simulink model "SLS_ChainModel_Sim"  (R2025a)
settings: Solver=VariableStepAuto  StartTime=0.0  StopTime=50  FixedStep=1e-3  RelTol=1e-3
values from neighbouring files (symbols this model uses):
  Phiu1 = full(Phiu{1})    [Distributed_Sim.m]
  Phiu2 = full(Phiu{2})    [Distributed_Sim.m]
  Phiu3 = full(Phiu{3})    [Distributed_Sim.m]
  Phiu4 = full(Phiu{4})    [Distributed_Sim.m]
  Phix1 = full(Phix{1})    [Distributed_Sim.m]
  Phix2 = full(Phix{2})    [Distributed_Sim.m]
  Phix3 = full(Phix{3})    [Distributed_Sim.m]
  Phix4 = full(Phix{4})    [Distributed_Sim.m]
  slsp1 = SLSPoles(1)    [Distributed_Sim.m]
  slsp2 = SLSPoles(2)    [Distributed_Sim.m]
  slsp3 = SLSPoles(3)    [Distributed_Sim.m]
  slsp4 = SLSPoles(4)    [Distributed_Sim.m]
  sysA = sys.A    [Distributed_Sim.m]    (also in Simple_Poles_Hinf.m = powersys.A; grid_model.mat = )
  sysB = sys.B2    [Distributed_Sim.m]    (also in Simple_Poles_Hinf.m = powersys.B2; grid_model.mat = )
undefined symbols (not defined in the file or in its folder): full
settings Model: Creator=johnd  LastModifiedBy=johnd
settings RTWCC: GPUComputeCapability=3.5

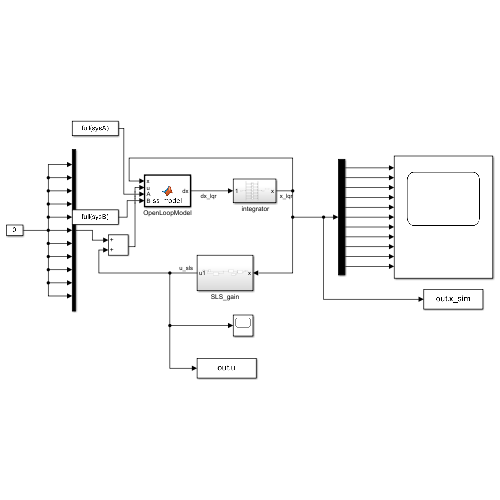
[thumbnail: Simulink's stored preview of the top-level diagram]
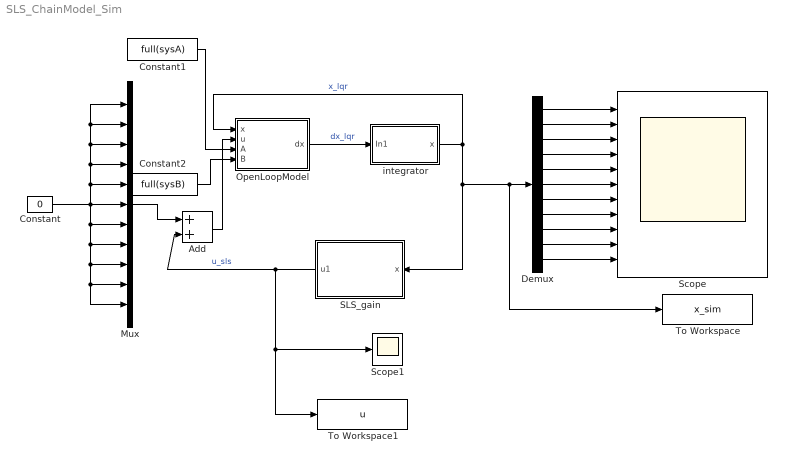
== system SLS_ChainModel_Sim ==
  " integrator" : Subsystem
  Add : Sum
  Constant : Constant  Value=0
  Constant1 : Constant  Value=full(sysA)
  Constant2 : Constant  Value=full(sysB)
  Demux : Demux  Outputs=11
  Mux : Mux  Inputs=11
  OpenLoopModel : MATLAB Function  TreatAsAtomicUnit=on
  SLS_gain : Subsystem
  Scope : Scope  NumInputPorts=11
      settings: ActiveDisplayYMinimum=-2.9E-35  ActiveDisplayYMaximum=3E-36
  Scope1 : Scope
      settings: ActiveDisplayYMinimum=-2.09753  ActiveDisplayYMaximum=0.3482
  To Workspace : ToWorkspace  VariableName=x_sim  SaveFormat=Timeseries  SampleTime=-1
  To Workspace1 : ToWorkspace  VariableName=u  SaveFormat=Timeseries  SampleTime=-1
  wires:
  OpenLoopModel/1(dx) -> " integrator"/1(In1)  "dx_lqr"
  " integrator"/1(x) -> SLS_gain/1(x), To Workspace/1, Demux/1, OpenLoopModel/1(x)  "x_lqr"
  Constant/1 -> Mux/6, Mux/7, Mux/8, Mux/9, Mux/10, Mux/11, Mux/5, Mux/4, Mux/3, Mux/2, Mux/1
  SLS_gain/1(u1) -> To Workspace1/1, Scope1/1, Add/2  "u_sls"
  Mux/1 -> Add/1
  Add/1 -> OpenLoopModel/2(u)
  Demux/1 -> Scope/1
  Demux/3 -> Scope/3
  Demux/2 -> Scope/2
  Demux/4 -> Scope/4
  Demux/5 -> Scope/5
  Demux/6 -> Scope/6
  Demux/7 -> Scope/7
  Demux/8 -> Scope/8
  Demux/9 -> Scope/9
  Demux/10 -> Scope/10
  Demux/11 -> Scope/11
  Constant1/1 -> OpenLoopModel/3(A)
  Constant2/1 -> OpenLoopModel/4(B)

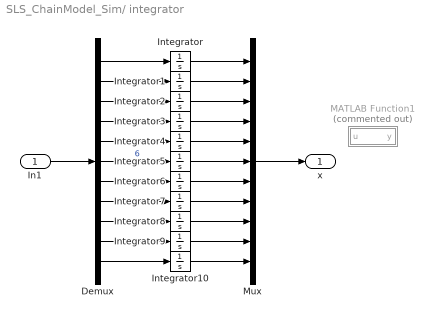
== system SLS_ChainModel_Sim/ integrator ==
  In1 : Inport
  Demux : Demux  Outputs=11
  Integrator{,1..4,6..10} (10 alike) : Integrator
  Integrator5 : Integrator  InitialCondition=1
  MATLAB Function1 : MATLAB Function  Commented=on  TreatAsAtomicUnit=on
  Mux : Mux  Inputs=11
  x : Outport
  wires:
  Demux/1 -> Integrator/1
  Demux/2 -> Integrator1/1
  Mux/1 -> x/1
  In1/1 -> Demux/1
  Demux/3 -> Integrator2/1
  Demux/4 -> Integrator3/1
  Demux/5 -> Integrator4/1
  Demux/6 -> Integrator5/1  "6"
  Demux/7 -> Integrator6/1
  Demux/8 -> Integrator7/1
  Demux/9 -> Integrator8/1
  Demux/10 -> Integrator9/1
  Demux/11 -> Integrator10/1
  Integrator/1 -> Mux/1
  Integrator1/1 -> Mux/2
  Integrator2/1 -> Mux/3
  Integrator3/1 -> Mux/4
  Integrator4/1 -> Mux/5
  Integrator5/1 -> Mux/6
  Integrator6/1 -> Mux/7
  Integrator7/1 -> Mux/8
  Integrator8/1 -> Mux/9
  Integrator9/1 -> Mux/10
  Integrator10/1 -> Mux/11

== system SLS_ChainModel_Sim/SLS_gain ==
  x : Inport
  Constant : Constant  Value=full(sysB)
  MATLAB Function : MATLAB Function  TreatAsAtomicUnit=on
  S*Phi_u(s)1 : Subsystem
  S*Phi_x(s) : Subsystem
  Subtract1 : Sum  Inputs=+-
  u1 : Outport
  wires:
  Subtract1/1 -> S*Phi_u(s)1/1(I), S*Phi_x(s)/1(v)  "v"
  x/1 -> Subtract1/1
  S*Phi_x(s)/1((s*phi_x(s)-I)) -> Subtract1/2
  S*Phi_u(s)1/1(s*phi_u(s)) -> MATLAB Function/1(u)
  MATLAB Function/1(y) -> u1/1
  Constant/1 -> MATLAB Function/2(B)

== system SLS_ChainModel_Sim/SLS_gain/S*Phi_u(s)1 ==
  note: This is for a 2-poles system
  I : Inport
  Add : Sum
  Pair1 : Subsystem
  Pair2 : Subsystem
  s*phi_u(s) : Outport
  wires:
  I/1 -> Pair2/1(u), Pair1/1(u)
  Pair1/1(s*phi_u(s)) -> Add/1
  Add/1 -> s*phi_u(s)/1
  Pair2/1(s*phi_u(s)) -> Add/2

== system SLS_ChainModel_Sim/SLS_gain/S*Phi_x(s) ==
  note: This is for a 2-poles system
  v : Inport
  Add : Sum
  Pair1 : Subsystem
  Pair2 : Subsystem
  (s*phi_x(s)-I) : Outport
  wires:
  v/1 -> Pair1/1(In1), Pair2/1(v)
  Pair1/1(Out1) -> Add/1
  Pair2/1(Out1) -> Add/2
  Add/1 -> (s*phi_x(s)-I)/1

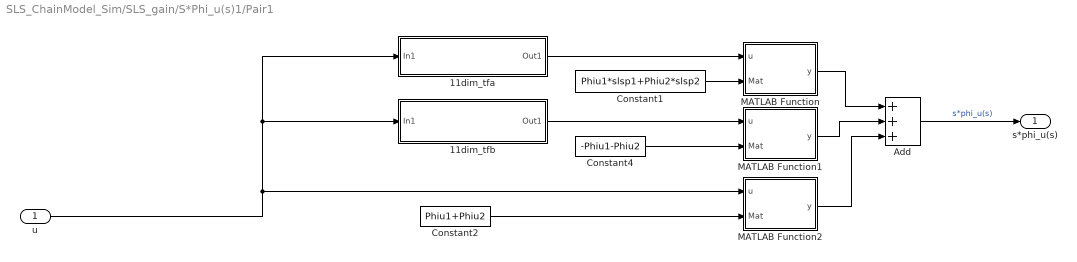
== system SLS_ChainModel_Sim/SLS_gain/S*Phi_u(s)1/Pair1 ==
  u : Inport
  11dim_tfa : Subsystem
  11dim_tfb : Subsystem
  Add : Sum  Inputs=+++
  Constant1 : Constant  Value=Phiu1*slsp1+Phiu2*slsp2  VectorParams1D=off
  Constant2 : Constant  Value=Phiu1+Phiu2
  Constant4 : Constant  Value=-Phiu1-Phiu2
  MATLAB Function : MATLAB Function  TreatAsAtomicUnit=on
  MATLAB Function1 : MATLAB Function  TreatAsAtomicUnit=on
  MATLAB Function2 : MATLAB Function  TreatAsAtomicUnit=on
  s*phi_u(s) : Outport
  wires:
  MATLAB Function/1(y) -> Add/1
  u/1 -> 11dim_tfb/1(In1), 11dim_tfa/1(In1), MATLAB Function2/1(u)
  11dim_tfa/1(Out1) -> MATLAB Function/1(u)
  MATLAB Function1/1(y) -> Add/2
  11dim_tfb/1(Out1) -> MATLAB Function1/1(u)
  MATLAB Function2/1(y) -> Add/3
  Constant1/1 -> MATLAB Function/2(Mat)
  Constant2/1 -> MATLAB Function2/2(Mat)
  Constant4/1 -> MATLAB Function1/2(Mat)
  Add/1 -> s*phi_u(s)/1  "s*phi_u(s)"

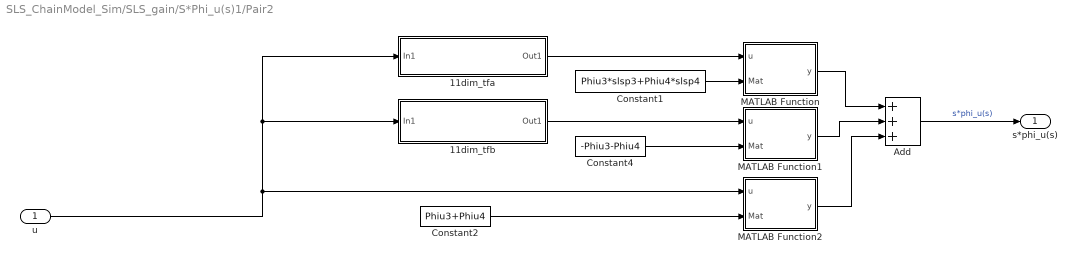
== system SLS_ChainModel_Sim/SLS_gain/S*Phi_u(s)1/Pair2 ==
  u : Inport
  11dim_tfa : Subsystem
  11dim_tfb : Subsystem
  Add : Sum  Inputs=+++
  Constant1 : Constant  Value=Phiu3*slsp3+Phiu4*slsp4  VectorParams1D=off
  Constant2 : Constant  Value=Phiu3+Phiu4
  Constant4 : Constant  Value=-Phiu3-Phiu4
  MATLAB Function : MATLAB Function  TreatAsAtomicUnit=on
  MATLAB Function1 : MATLAB Function  TreatAsAtomicUnit=on
  MATLAB Function2 : MATLAB Function  TreatAsAtomicUnit=on
  s*phi_u(s) : Outport
  wires:
  Add/1 -> s*phi_u(s)/1  "s*phi_u(s)"
  Constant4/1 -> MATLAB Function1/2(Mat)
  Constant2/1 -> MATLAB Function2/2(Mat)
  Constant1/1 -> MATLAB Function/2(Mat)
  MATLAB Function2/1(y) -> Add/3
  11dim_tfb/1(Out1) -> MATLAB Function1/1(u)
  MATLAB Function1/1(y) -> Add/2
  11dim_tfa/1(Out1) -> MATLAB Function/1(u)
  u/1 -> MATLAB Function2/1(u), 11dim_tfa/1(In1), 11dim_tfb/1(In1)
  MATLAB Function/1(y) -> Add/1

== system SLS_ChainModel_Sim/SLS_gain/S*Phi_x(s)/Pair1 ==
  In1 : Inport
  11dim_tfa : Subsystem
  11dim_tfb : Subsystem
  Add : Sum
  Constant1 : Constant  Value=Phix1*slsp1+Phix2*slsp2
  Constant4 : Constant  Value=-Phix1-Phix2
  MATLAB Function : MATLAB Function  TreatAsAtomicUnit=on
  MATLAB Function1 : MATLAB Function  TreatAsAtomicUnit=on
  Out1 : Outport
  wires:
  Add/1 -> Out1/1
  MATLAB Function/1(y) -> Add/1
  11dim_tfb/1(Out1) -> MATLAB Function1/1(u)
  In1/1 -> 11dim_tfa/1(In1), 11dim_tfb/1(In1)
  11dim_tfa/1(Out1) -> MATLAB Function/1(u)
  MATLAB Function1/1(y) -> Add/2
  Constant1/1 -> MATLAB Function/2(Mat)
  Constant4/1 -> MATLAB Function1/2(Mat)

== system SLS_ChainModel_Sim/SLS_gain/S*Phi_x(s)/Pair2 ==
  v : Inport
  11dim_tfa : Subsystem
  11dim_tfb : Subsystem
  Add : Sum
  Constant1 : Constant  Value=Phix3*slsp3+Phix4*slsp4
  Constant4 : Constant  Value=-Phix3-Phix4
  MATLAB Function : MATLAB Function  TreatAsAtomicUnit=on
  MATLAB Function1 : MATLAB Function  TreatAsAtomicUnit=on
  Out1 : Outport
  wires:
  Constant4/1 -> MATLAB Function1/2(Mat)
  Constant1/1 -> MATLAB Function/2(Mat)
  MATLAB Function1/1(y) -> Add/2
  11dim_tfa/1(Out1) -> MATLAB Function/1(u)
  v/1 -> 11dim_tfb/1(In1), 11dim_tfa/1(In1)
  11dim_tfb/1(Out1) -> MATLAB Function1/1(u)
  MATLAB Function/1(y) -> Add/1
  Add/1 -> Out1/1

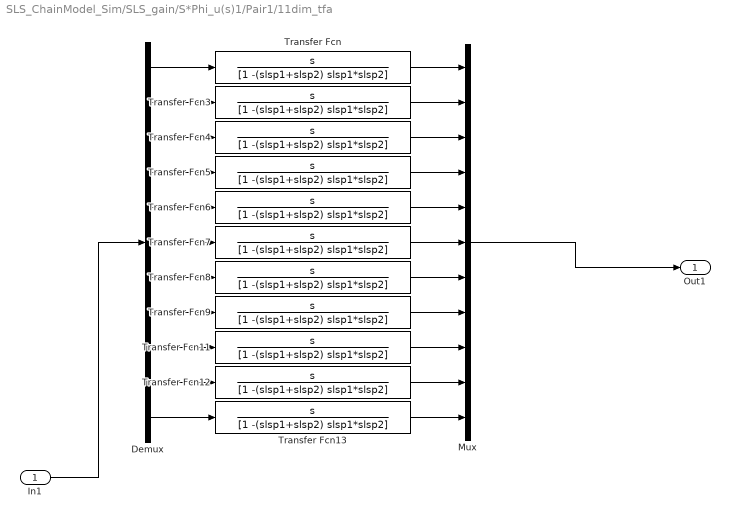
== system SLS_ChainModel_Sim/SLS_gain/S*Phi_u(s)1/Pair1/11dim_tfa ==
  In1 : Inport
  Demux : Demux  Outputs=11
  Mux : Mux  Inputs=11
  Transfer Fcn{,3..9,11..13} (11 alike) : TransferFcn  Numerator=[0 1 0]  Denominator=[1 -(slsp1+slsp2) slsp1*slsp2]
  Out1 : Outport
  wires:
  Transfer Fcn12/1 -> Mux/10
  Demux/7 -> Transfer Fcn8/1
  Transfer Fcn7/1 -> Mux/6
  Demux/4 -> Transfer Fcn5/1
  Demux/2 -> Transfer Fcn3/1
  Demux/9 -> Transfer Fcn11/1
  In1/1 -> Demux/1
  Transfer Fcn9/1 -> Mux/8
  Demux/10 -> Transfer Fcn12/1
  Demux/6 -> Transfer Fcn7/1
  Demux/11 -> Transfer Fcn13/1
  Demux/8 -> Transfer Fcn9/1
  Transfer Fcn11/1 -> Mux/9
  Transfer Fcn5/1 -> Mux/4
  Transfer Fcn3/1 -> Mux/2
  Transfer Fcn4/1 -> Mux/3
  Transfer Fcn6/1 -> Mux/5
  Demux/5 -> Transfer Fcn6/1
  Mux/1 -> Out1/1
  Demux/3 -> Transfer Fcn4/1
  Transfer Fcn8/1 -> Mux/7
  Transfer Fcn13/1 -> Mux/11
  Demux/1 -> Transfer Fcn/1
  Transfer Fcn/1 -> Mux/1

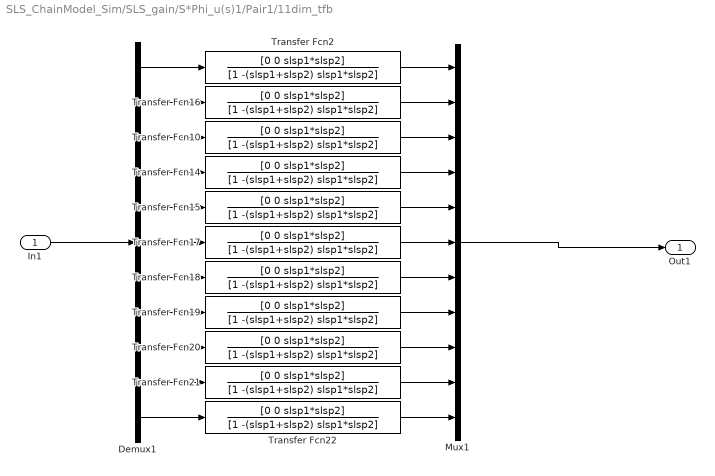
== system SLS_ChainModel_Sim/SLS_gain/S*Phi_u(s)1/Pair1/11dim_tfb ==
  In1 : Inport
  Demux1 : Demux  Outputs=11
  Mux1 : Mux  Inputs=11
  Transfer Fcn{2,10,14..22} (11 alike) : TransferFcn  Numerator=[0 0 slsp1*slsp2]  Denominator=[1 -(slsp1+slsp2) slsp1*slsp2]
  Out1 : Outport
  wires:
  Transfer Fcn20/1 -> Mux1/9
  Demux1/8 -> Transfer Fcn19/1
  Transfer Fcn18/1 -> Mux1/7
  Demux1/7 -> Transfer Fcn18/1
  Transfer Fcn19/1 -> Mux1/8
  Demux1/11 -> Transfer Fcn22/1
  Demux1/4 -> Transfer Fcn14/1
  Transfer Fcn16/1 -> Mux1/2
  Demux1/3 -> Transfer Fcn10/1
  Transfer Fcn10/1 -> Mux1/3
  Demux1/2 -> Transfer Fcn16/1
  Demux1/9 -> Transfer Fcn20/1
  Demux1/10 -> Transfer Fcn21/1
  Transfer Fcn2/1 -> Mux1/1
  Transfer Fcn22/1 -> Mux1/11
  Demux1/1 -> Transfer Fcn2/1
  Demux1/5 -> Transfer Fcn15/1
  In1/1 -> Demux1/1
  Mux1/1 -> Out1/1
  Transfer Fcn15/1 -> Mux1/5
  Demux1/6 -> Transfer Fcn17/1
  Transfer Fcn17/1 -> Mux1/6
  Transfer Fcn14/1 -> Mux1/4
  Transfer Fcn21/1 -> Mux1/10

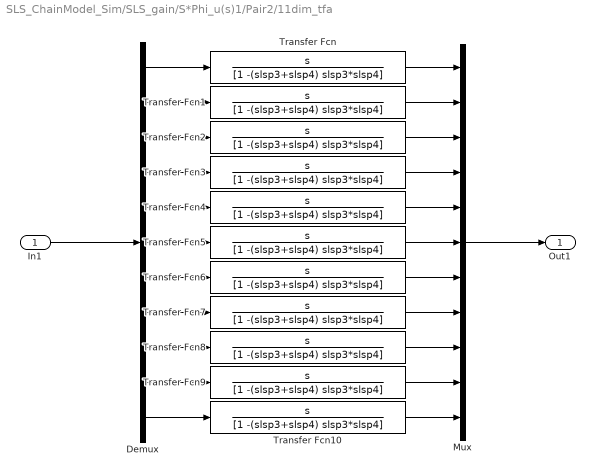
== system SLS_ChainModel_Sim/SLS_gain/S*Phi_u(s)1/Pair2/11dim_tfa ==
  In1 : Inport
  Demux : Demux  Outputs=11
  Mux : Mux  Inputs=11
  Transfer Fcn{,1..10} (11 alike) : TransferFcn  Numerator=[0 1 0]  Denominator=[1 -(slsp3+slsp4) slsp3*slsp4]
  Out1 : Outport
  wires:
  Transfer Fcn/1 -> Mux/1
  Demux/1 -> Transfer Fcn/1
  Transfer Fcn10/1 -> Mux/11
  Transfer Fcn6/1 -> Mux/7
  Demux/3 -> Transfer Fcn2/1
  Mux/1 -> Out1/1
  Demux/5 -> Transfer Fcn4/1
  Transfer Fcn4/1 -> Mux/5
  Transfer Fcn2/1 -> Mux/3
  Transfer Fcn1/1 -> Mux/2
  Transfer Fcn3/1 -> Mux/4
  Transfer Fcn8/1 -> Mux/9
  Demux/8 -> Transfer Fcn7/1
  Demux/11 -> Transfer Fcn10/1
  Demux/6 -> Transfer Fcn5/1
  Demux/10 -> Transfer Fcn9/1
  Transfer Fcn7/1 -> Mux/8
  In1/1 -> Demux/1
  Demux/9 -> Transfer Fcn8/1
  Demux/2 -> Transfer Fcn1/1
  Demux/4 -> Transfer Fcn3/1
  Transfer Fcn5/1 -> Mux/6
  Demux/7 -> Transfer Fcn6/1
  Transfer Fcn9/1 -> Mux/10

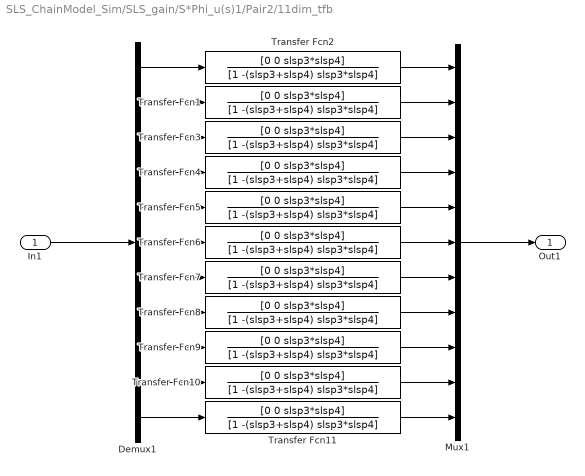
== system SLS_ChainModel_Sim/SLS_gain/S*Phi_u(s)1/Pair2/11dim_tfb ==
  In1 : Inport
  Demux1 : Demux  Outputs=11
  Mux1 : Mux  Inputs=11
  Transfer Fcn{1..11} (11 alike) : TransferFcn  Numerator=[0 0 slsp3*slsp4]  Denominator=[1 -(slsp3+slsp4) slsp3*slsp4]
  Out1 : Outport
  wires:
  Transfer Fcn10/1 -> Mux1/10
  Transfer Fcn4/1 -> Mux1/4
  Transfer Fcn6/1 -> Mux1/6
  Demux1/6 -> Transfer Fcn6/1
  Transfer Fcn5/1 -> Mux1/5
  Mux1/1 -> Out1/1
  In1/1 -> Demux1/1
  Demux1/5 -> Transfer Fcn5/1
  Demux1/1 -> Transfer Fcn2/1
  Transfer Fcn11/1 -> Mux1/11
  Transfer Fcn2/1 -> Mux1/1
  Demux1/10 -> Transfer Fcn10/1
  Demux1/9 -> Transfer Fcn9/1
  Demux1/2 -> Transfer Fcn1/1
  Transfer Fcn3/1 -> Mux1/3
  Demux1/3 -> Transfer Fcn3/1
  Transfer Fcn1/1 -> Mux1/2
  Demux1/4 -> Transfer Fcn4/1
  Demux1/11 -> Transfer Fcn11/1
  Transfer Fcn8/1 -> Mux1/8
  Demux1/7 -> Transfer Fcn7/1
  Transfer Fcn7/1 -> Mux1/7
  Demux1/8 -> Transfer Fcn8/1
  Transfer Fcn9/1 -> Mux1/9

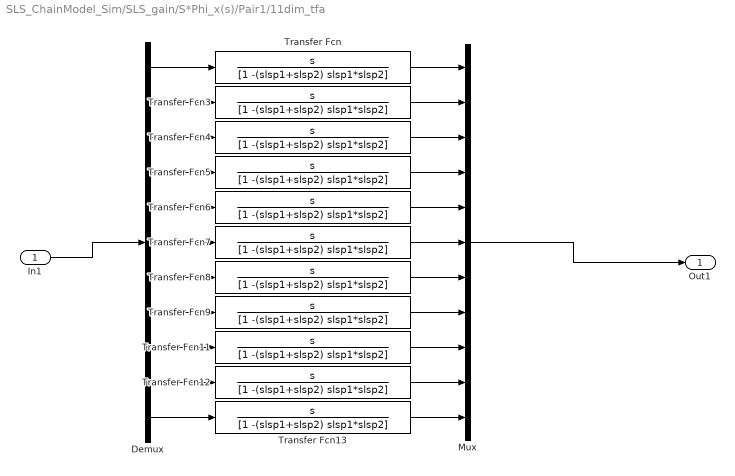
== system SLS_ChainModel_Sim/SLS_gain/S*Phi_x(s)/Pair1/11dim_tfa ==
  In1 : Inport
  Demux : Demux  Outputs=11
  Mux : Mux  Inputs=11
  Transfer Fcn{,3..9,11..13} (11 alike) : TransferFcn  Numerator=[0 1 0]  Denominator=[1 -(slsp1+slsp2) slsp1*slsp2]
  Out1 : Outport
  wires:
  Transfer Fcn13/1 -> Mux/11
  Transfer Fcn3/1 -> Mux/2
  Demux/5 -> Transfer Fcn6/1
  Demux/1 -> Transfer Fcn/1
  Transfer Fcn4/1 -> Mux/3
  Demux/7 -> Transfer Fcn8/1
  Transfer Fcn8/1 -> Mux/7
  Transfer Fcn6/1 -> Mux/5
  Transfer Fcn/1 -> Mux/1
  Demux/2 -> Transfer Fcn3/1
  Demux/8 -> Transfer Fcn9/1
  Transfer Fcn11/1 -> Mux/9
  Demux/3 -> Transfer Fcn4/1
  Transfer Fcn12/1 -> Mux/10
  Demux/11 -> Transfer Fcn13/1
  Transfer Fcn7/1 -> Mux/6
  Transfer Fcn9/1 -> Mux/8
  Demux/6 -> Transfer Fcn7/1
  Demux/4 -> Transfer Fcn5/1
  Demux/10 -> Transfer Fcn12/1
  Mux/1 -> Out1/1
  Transfer Fcn5/1 -> Mux/4
  Demux/9 -> Transfer Fcn11/1
  In1/1 -> Demux/1

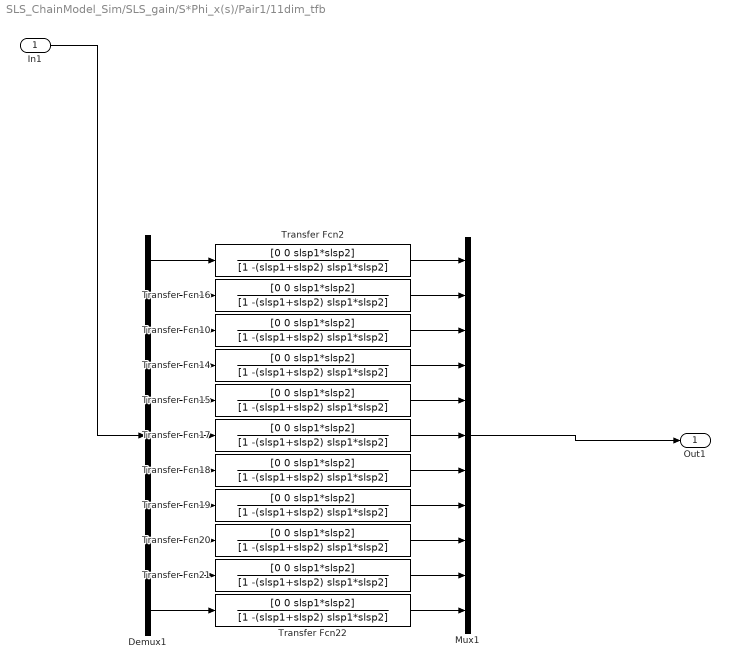
== system SLS_ChainModel_Sim/SLS_gain/S*Phi_x(s)/Pair1/11dim_tfb ==
  In1 : Inport
  Demux1 : Demux  Outputs=11
  Mux1 : Mux  Inputs=11
  Transfer Fcn{2,10,14..22} (11 alike) : TransferFcn  Numerator=[0 0 slsp1*slsp2]  Denominator=[1 -(slsp1+slsp2) slsp1*slsp2]
  Out1 : Outport
  wires:
  Transfer Fcn15/1 -> Mux1/5
  Transfer Fcn17/1 -> Mux1/6
  Transfer Fcn21/1 -> Mux1/10
  Demux1/6 -> Transfer Fcn17/1
  Demux1/1 -> Transfer Fcn2/1
  Transfer Fcn2/1 -> Mux1/1
  Demux1/11 -> Transfer Fcn22/1
  Demux1/5 -> Transfer Fcn15/1
  Transfer Fcn22/1 -> Mux1/11
  Demux1/10 -> Transfer Fcn21/1
  Demux1/2 -> Transfer Fcn16/1
  Transfer Fcn16/1 -> Mux1/2
  Demux1/9 -> Transfer Fcn20/1
  Transfer Fcn20/1 -> Mux1/9
  Demux1/7 -> Transfer Fcn18/1
  Transfer Fcn18/1 -> Mux1/7
  Transfer Fcn14/1 -> Mux1/4
  Demux1/4 -> Transfer Fcn14/1
  Transfer Fcn10/1 -> Mux1/3
  Demux1/3 -> Transfer Fcn10/1
  Demux1/8 -> Transfer Fcn19/1
  Transfer Fcn19/1 -> Mux1/8
  In1/1 -> Demux1/1
  Mux1/1 -> Out1/1

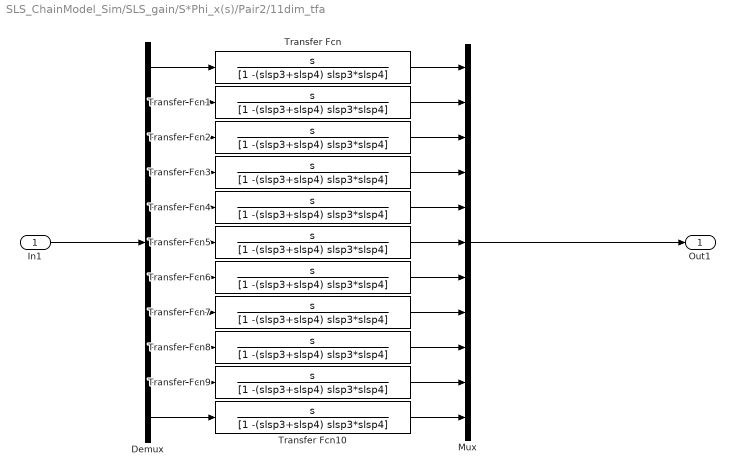
== system SLS_ChainModel_Sim/SLS_gain/S*Phi_x(s)/Pair2/11dim_tfa ==
  In1 : Inport
  Demux : Demux  Outputs=11
  Mux : Mux  Inputs=11
  Transfer Fcn{,1..10} (11 alike) : TransferFcn  Numerator=[0 1 0]  Denominator=[1 -(slsp3+slsp4) slsp3*slsp4]
  Out1 : Outport
  wires:
  In1/1 -> Demux/1
  Demux/9 -> Transfer Fcn8/1
  Transfer Fcn3/1 -> Mux/4
  Mux/1 -> Out1/1
  Demux/10 -> Transfer Fcn9/1
  Demux/4 -> Transfer Fcn3/1
  Demux/6 -> Transfer Fcn5/1
  Transfer Fcn7/1 -> Mux/8
  Transfer Fcn5/1 -> Mux/6
  Demux/11 -> Transfer Fcn10/1
  Transfer Fcn9/1 -> Mux/10
  Demux/3 -> Transfer Fcn2/1
  Transfer Fcn8/1 -> Mux/9
  Demux/8 -> Transfer Fcn7/1
  Demux/2 -> Transfer Fcn1/1
  Transfer Fcn/1 -> Mux/1
  Transfer Fcn4/1 -> Mux/5
  Transfer Fcn6/1 -> Mux/7
  Demux/7 -> Transfer Fcn6/1
  Transfer Fcn2/1 -> Mux/3
  Demux/1 -> Transfer Fcn/1
  Demux/5 -> Transfer Fcn4/1
  Transfer Fcn1/1 -> Mux/2
  Transfer Fcn10/1 -> Mux/11

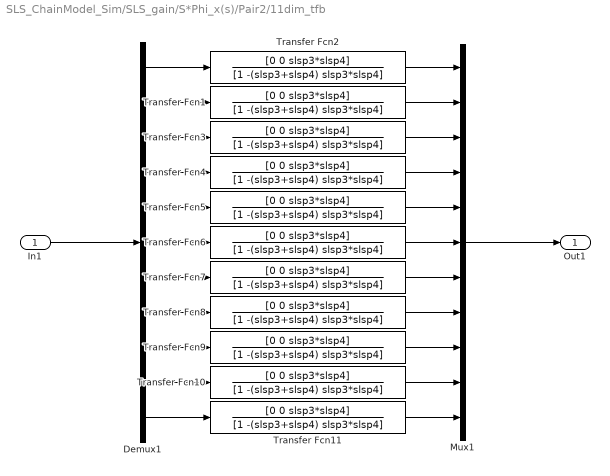
== system SLS_ChainModel_Sim/SLS_gain/S*Phi_x(s)/Pair2/11dim_tfb ==
  In1 : Inport
  Demux1 : Demux  Outputs=11
  Mux1 : Mux  Inputs=11
  Transfer Fcn{1..11} (11 alike) : TransferFcn  Numerator=[0 0 slsp3*slsp4]  Denominator=[1 -(slsp3+slsp4) slsp3*slsp4]
  Out1 : Outport
  wires:
  Mux1/1 -> Out1/1
  In1/1 -> Demux1/1
  Transfer Fcn8/1 -> Mux1/8
  Demux1/8 -> Transfer Fcn8/1
  Demux1/3 -> Transfer Fcn3/1
  Transfer Fcn3/1 -> Mux1/3
  Demux1/4 -> Transfer Fcn4/1
  Transfer Fcn4/1 -> Mux1/4
  Transfer Fcn7/1 -> Mux1/7
  Demux1/7 -> Transfer Fcn7/1
  Transfer Fcn9/1 -> Mux1/9
  Demux1/9 -> Transfer Fcn9/1
  Transfer Fcn1/1 -> Mux1/2
  Demux1/2 -> Transfer Fcn1/1
  Demux1/10 -> Transfer Fcn10/1
  Transfer Fcn11/1 -> Mux1/11
  Demux1/5 -> Transfer Fcn5/1
  Demux1/11 -> Transfer Fcn11/1
  Transfer Fcn2/1 -> Mux1/1
  Demux1/1 -> Transfer Fcn2/1
  Demux1/6 -> Transfer Fcn6/1
  Transfer Fcn10/1 -> Mux1/10
  Transfer Fcn6/1 -> Mux1/6
  Transfer Fcn5/1 -> Mux1/5

== matlab function SLS_ChainModel_Sim/SLS_gain/S*Phi_u(s)1/Pair2/MATLAB Function2 ==
  data: u input; Mat input; y output
function y = leftMult(u,Mat)

y = real(Mat)*u;

== matlab function SLS_ChainModel_Sim/SLS_gain/MATLAB Function ==
  data: u input; y output; B input
function y = fcn(u,B)

y = B*u;

== matlab function SLS_ChainModel_Sim/SLS_gain/S*Phi_u(s)1/Pair1/MATLAB Function ==
  data: u input; Mat input; y output
function y = leftMult(u,Mat)

y = real(Mat)*u;

== matlab function SLS_ChainModel_Sim/OpenLoopModel ==
  data: x input; u input; dx output; A input; B input
function dx = ss_model(x,u,A,B)
% A = [0.6000    0.4000         0         0         0         0         0         0         0         0         0
%     0.4000    0.6000    0.4000         0         0         0         0         0         0         0         0
%          0    0.4000    0.6000    0.4000         0         0         0         0         0         0         0
%          0         0    0.4000    0.6000    0.4000         0         0         0         0         0         0
%          0         0         0    0.4000    0.6000    0.4000         0         0         0         0         0
%          0         0         0         0    0.4000    0.6000    0.4000         0         0         0         0
%          0         0         0         0         0    0.4000    0.6000    0.4000         0         0         0
%          0         0         0         0         0         0    0.4000    0.6000    0.4000         0         0
%          0         0         0         0         0         0         0    0.4000    0.6000    0.4000         0
%          0         0         0         0         0         0         0         0    0.4000    0.6000    0.4000
%          0         0         0         0         0         0         0         0         0    0.4000    0.6000];
% B = [1     0     0     0     0     0     0     0     0     0     0
%      0     1     0     0     0     0     0     0     0     0     0
%      0     0     1     0     0     0     0     0     0     0     0
%      0     0     0     1     0     0     0     0     0     0     0
%      0     0     0     0     1     0     0     0     0     0     0
%      0     0     0     0     0     1     0     0     0     0     0
%      0     0     0     0     0     0     1     0     0     0     0
%      0     0     0     0     0     0     0     1     0     0     0
%      0     0     0     0     0     0     0     0     1     0     0
%      0     0     0     0     0     0     0     0     0     1     0
%      0     0     0     0     0     0     0     0     0     0     1];

dx = A*x+B*u;

== matlab function SLS_ChainModel_Sim/SLS_gain/S*Phi_u(s)1/Pair1/MATLAB Function1 ==
  data: u input; Mat input; y output
function y = leftMult(u,Mat)

y = real(Mat)*u;

== matlab function SLS_ChainModel_Sim/SLS_gain/S*Phi_u(s)1/Pair1/MATLAB Function2 ==
  data: u input; Mat input; y output
function y = leftMult(u,Mat)

y = real(Mat)*u;

== matlab function SLS_ChainModel_Sim/SLS_gain/S*Phi_x(s)/Pair1/MATLAB Function ==
  data: u input; Mat input; y output
function y = leftMult(u,Mat)

y = real(Mat)*u;

== matlab function SLS_ChainModel_Sim/SLS_gain/S*Phi_x(s)/Pair1/MATLAB Function1 ==
  data: u input; Mat input; y output
function y = leftMult(u,Mat)

y = real(Mat)*u;

== matlab function SLS_ChainModel_Sim/ integrator/MATLAB Function1 ==
  data: u input; y output
function y = round(u)

if abs(u) > 1e-16
y = u;
else
    y = 0;
end

== matlab function SLS_ChainModel_Sim/SLS_gain/S*Phi_x(s)/Pair2/MATLAB Function ==
  data: u input; Mat input; y output
function y = leftMult(u,Mat)

y = real(Mat)*u;

== matlab function SLS_ChainModel_Sim/SLS_gain/S*Phi_x(s)/Pair2/MATLAB Function1 ==
  data: u input; Mat input; y output
function y = leftMult(u,Mat)

y = real(Mat)*u;

== matlab function SLS_ChainModel_Sim/SLS_gain/S*Phi_u(s)1/Pair2/MATLAB Function ==
  data: u input; Mat input; y output
function y = leftMult(u,Mat)

y = real(Mat)*u;

== matlab function SLS_ChainModel_Sim/SLS_gain/S*Phi_u(s)1/Pair2/MATLAB Function1 ==
  data: u input; Mat input; y output
function y = leftMult(u,Mat)

y = real(Mat)*u;
